simulink model "GuytonModel1986All_R2015a"  (R2015a)
settings: Solver=ode15s  StartTime=0  StopTime=383040  FixedStep=0.03  MaxStep=360  RelTol=1e-3
libraries: simulink x3
(part 3 of 5)

== system GuytonModel1986All_R2015a/Macula densa ==
  note: MACULA DENSA
  note: FNA
  note: NAPT1
  note: DAMPING
  CNA : Inport
  GFN : Inport  Port=2
  Constant1 : Constant
  Constant2 : Constant
  Constant3 : Constant
  Constant7 : Constant  Value=0.057
  GF2 : Constant  Value=0.1
  Integrator1 : Integrator  InitialConditionSource=external
  Product{2..3,7,15} (4 alike) : Product  SaturateOnIntegerOverflow=on  RndMeth=Zero  InputSameDT=on  OutDataTypeStr=Inherit: Same as first input
  RNAUGN : Constant  Value=5
  Sum3 : Sum  SaturateOnIntegerOverflow=on  InputSameDT=on  OutDataTypeStr=Inherit: Same as first input
  Sum30 : Sum  Inputs=+-  SaturateOnIntegerOverflow=on  InputSameDT=on  OutDataTypeStr=Inherit: Same as first input
  Sum9 : Sum  Inputs=-+  SaturateOnIntegerOverflow=on  InputSameDT=on  OutDataTypeStr=Inherit: Same as first input
  "upper limit 10 lower limit 0.3 " : Saturate  UpperLimit=10  LowerLimit=0.3  LinearizeAsGain=off
  upper limit 3.0 lower limit 0.1 : Saturate  UpperLimit=3  LowerLimit=0.1  LinearizeAsGain=off
  NAPT1 : Outport
  RNAUG1 : Outport  Port=2
  wires:
  Product15/1 -> Product3/1
  GFN/1 -> Product15/2
  CNA/1 -> Product15/1  "CNA"
  Constant7/1 -> Product3/2
  Product3/1 -> upper limit 3.0 lower limit 0.1/1  "NAPT"
  Constant1/1 -> Integrator1/2
  upper limit 3.0 lower limit 0.1/1 -> Sum9/2  "NAPT"
  GF2/1 -> Product7/2
  Sum9/1 -> Product7/1
  Product7/1 -> Integrator1/1
  Integrator1/1 -> Sum30/1, NAPT1/1, Sum9/1  "NAPT1"
  Constant2/1 -> Sum30/2
  Sum30/1 -> Product2/2
  RNAUGN/1 -> Product2/1
  Product2/1 -> Sum3/1
  Constant3/1 -> Sum3/2
  Sum3/1 -> "upper limit 10 lower limit 0.3 "/1
  "upper limit 10 lower limit 0.3 "/1 -> RNAUG1/1

== system GuytonModel1986All_R2015a/Muscle Local Blood Flow Control  ==
  note: Long term autoregulation
  note: Short term autoregulation
  note: AMM1
  note: if (POE<0.05) {POE=0.05}
  note: ARM
  note: Muscle Local Blood Flow Contro
  PMO : Inport
  A4K : Constant  Value=10
  A4K2 : Constant  Value=10000
  POK{1,4..5,10} (4 alike) : Constant
  POK15 : Constant  Value=0.3
  POK3 : Constant  Value=0.05
  POM : Constant  Value=0.2
  POM2 : Constant  Value=16
  PORM : Constant  Value=8
  Product : Product  SaturateOnIntegerOverflow=on  RndMeth=Zero  InputSameDT=on  OutDataTypeStr=Inherit: Same as first input
  Product1 : Product  Inputs=*/  SaturateOnIntegerOverflow=on  RndMeth=Zero  InputSameDT=on  OutDataTypeStr=Inherit: Same as first input
  Product5 : Product  SaturateOnIntegerOverflow=on  RndMeth=Zero  InputSameDT=on  OutDataTypeStr=Inherit: Same as first input
  Product7 : Product  Inputs=*/  SaturateOnIntegerOverflow=on  RndMeth=Zero  InputSameDT=on  OutDataTypeStr=Inherit: Same as first input
  Product8 : Product  SaturateOnIntegerOverflow=on  RndMeth=Zero  InputSameDT=on  OutDataTypeStr=Inherit: Same as first input
  Sum1 : Sum  Inputs=++|  SaturateOnIntegerOverflow=on  InputSameDT=on  OutDataTypeStr=Inherit: Same as first input
  Sum3 : Sum  Inputs=-+|  SaturateOnIntegerOverflow=on  InputSameDT=on  OutDataTypeStr=Inherit: Same as first input
  Sum7 : Sum  Inputs=+-  SaturateOnIntegerOverflow=on  InputSameDT=on  OutDataTypeStr=Inherit: Same as first input
  Sum8 : Sum  Inputs=++|  SaturateOnIntegerOverflow=on  InputSameDT=on  OutDataTypeStr=Inherit: Same as first input
  Sum9 : Sum  Inputs=-+|  SaturateOnIntegerOverflow=on  InputSameDT=on  OutDataTypeStr=Inherit: Same as first input
  Switch3 : Switch  Threshold=0.3  SaturateOnIntegerOverflow=on  InputSameDT=on
  Switch5 : Switch  Threshold=0.05  SaturateOnIntegerOverflow=on  InputSameDT=on
  integrator POB1 : Integrator  InitialConditionSource=external  InitialCondition=0.6577
  integrator POB4 : Integrator  InitialConditionSource=external  InitialCondition=0.6577
  " AMM" : Outport
  wires:
  Sum7/1 -> Product5/1, Product/1  "PDO"
  Sum8/1 -> Switch3/1, Switch3/2  "POF"
  Switch3/1 -> Sum9/2
  POK15/1 -> Switch3/3
  A4K2/1 -> Product7/2
  Sum9/1 -> Product7/1
  Product7/1 -> integrator POB4/1  "(POF-AMM2)/A4K2"
  POK10/1 -> integrator POB4/2
  integrator POB4/1 -> Sum9/1, Product8/1  "AMM2"
  POK5/1 -> Sum8/1
  Product5/1 -> Sum8/2
  POM2/1 -> Product5/2
  Product8/1 -> " AMM"/1
  Product1/1 -> integrator POB1/1  "(POE-AMM1)/A4K"
  A4K/1 -> Product1/2
  Sum3/1 -> Product1/1
  integrator POB1/1 -> Product8/2, Sum3/1  "AMM1"
  Switch5/1 -> Sum3/2  "POE"
  POK4/1 -> integrator POB1/2
  POK3/1 -> Switch5/3
  Sum1/1 -> Switch5/1, Switch5/2  "POE"
  POK1/1 -> Sum1/1
  Product/1 -> Sum1/2
  POM/1 -> Product/2
  PORM/1 -> Sum7/2
  PMO/1 -> Sum7/1

== system GuytonModel1986All_R2015a/Myogenic Autoregulation ==
  note: PA+PC
  note: PDIFF
  note: PADAPT
  note: PDIFF
  note: PADAPT
  note: Myogenic Autoregulation
  PA : Inport
  PC : Inport  Port=2
  MYOGTAU : Inport  Port=3
  TENSGN : Inport  Port=4
  Add25 : Sum
  Constant1 : Constant  Value=117
  Derivative : Derivative
  Integrator1 : Integrator  InitialConditionSource=external
  RAPDel=RAP-RAPAdp : Sum  Inputs=+-  SaturateOnIntegerOverflow=on  InputSameDT=on  OutDataTypeStr=Inherit: Same as first input
  RAPdot=RAPdel/AffTau : Product  Inputs=*/  SaturateOnIntegerOverflow=on  InputSameDT=on  OutDataTypeStr=Inherit: Same as first input
  RAPdot=RAPdel/AffTau1 : Product  Inputs=*/  SaturateOnIntegerOverflow=on  InputSameDT=on  OutDataTypeStr=Inherit: Same as first input
  RAPdot=RAPdel/AffTau2 : Product  Inputs=**  SaturateOnIntegerOverflow=on  InputSameDT=on  OutDataTypeStr=Inherit: Same as first input
  "[X,Y,Slope...]  - data from Coleman (1992)" : Constant  Value=[-30.0,1.5,0.0,0.0,1.0,-0.02,80.0,0.5,0.0]
  function MyogenResp(PDIFF) - spline interpolation : Subsystem  TreatAsAtomicUnit=on
      mask help: CURVILINEAR
      mask Help: Interpolates function value using  linear (if x<=0 or x>=x2) or cubic spline (if x0>x<x2) interpolation
      mask Display:
      | disp('C U R V I L I N E A R\n\nInterpolates function value \nusing  linear (if x<=0 or x>=x2)
      | \nor cubic spline (if x0>x<x2) interpolation\n\nINPUTS :\nx  -  value of independent variable\n xySlope - vector of coordinates and slope of 3 knots:\n[x0, y0, slope0,\n n1, y1, slope1,\n x2, y2, slope2]\n\nOUTPUTS :\ny - interpolated function value')
  MYOGRS : Outport
  wires:
  Constant1/1 -> Integrator1/2
  RAPdot=RAPdel/AffTau2/1 -> function MyogenResp(PDIFF) - spline interpolation/1(x)
  Derivative/1 -> RAPdot=RAPdel/AffTau2/1
  RAPdot=RAPdel/AffTau1/1 -> MYOGRS/1
  MYOGTAU/1 -> RAPdot=RAPdel/AffTau2/2, RAPdot=RAPdel/AffTau/2  "MYOGTAU"
  Integrator1/1 -> Derivative/1, RAPDel=RAP-RAPAdp/2
  RAPDel=RAP-RAPAdp/1 -> RAPdot=RAPdel/AffTau/1  "RAPDel"
  "[X,Y,Slope...]  - data from Coleman (1992)"/1 -> function MyogenResp(PDIFF) - spline interpolation/2(xySlope)
  RAPdot=RAPdel/AffTau/1 -> Integrator1/1  "DPADAPT"
  PC/1 -> Add25/2
  PA/1 -> Add25/1
  Add25/1 -> RAPDel=RAP-RAPAdp/1
  TENSGN/1 -> RAPdot=RAPdel/AffTau1/1
  function MyogenResp(PDIFF) - spline interpolation/1(y) -> RAPdot=RAPdel/AffTau1/2

== system GuytonModel1986All_R2015a/Myogenic Autoregulation of Afferent Arteriole ==
  note: MYOGENIC AUTOREGULATION IN KIDNEY
  note: PAR
  note: PADAPT
  note: PDIFF
  note: PADAPT
  PAR : Inport
  MYOGTAU : Inport  Port=2
  TENSGN : Inport  Port=3
  Constant1 : Constant  Value=100
  Integrator1 : Integrator  InitialConditionSource=external
  RAPDel=RAP-RAPAdp : Sum  Inputs=+-  SaturateOnIntegerOverflow=on  InputSameDT=on  OutDataTypeStr=Inherit: Same as first input
  RAPdot=RAPdel/AffTau : Product  Inputs=*/  SaturateOnIntegerOverflow=on  InputSameDT=on  OutDataTypeStr=Inherit: Same as first input
  RAPdot=RAPdel/AffTau1 : Product  Inputs=*/  SaturateOnIntegerOverflow=on  InputSameDT=on  OutDataTypeStr=Inherit: Same as first input
  "[X,Y,Slope...]  - data from Coleman (1992)" : Constant  Value=[-30.0,1.5,0.0,0.0,1.0,-0.02,80.0,0.5,0.0]
  function MyogenResp(PDIFF) - spline interpolation : Subsystem  TreatAsAtomicUnit=on
      mask help: CURVILINEAR
      mask Help: Interpolates function value using  linear (if x<=0 or x>=x2) or cubic spline (if x0>x<x2) interpolation
      mask Display:
      | disp('C U R V I L I N E A R\n\nInterpolates function value \nusing  linear (if x<=0 or x>=x2)
      | \nor cubic spline (if x0>x<x2) interpolation\n\nINPUTS :\nx  -  value of independent variable\n xySlope - vector of coordinates and slope of 3 knots:\n[x0, y0, slope0,\n n1, y1, slope1,\n x2, y2, slope2]\n\nOUTPUTS :\ny - interpolated function value')
  MYOGRSAA : Outport
  wires:
  Constant1/1 -> Integrator1/2
  RAPdot=RAPdel/AffTau1/1 -> MYOGRSAA/1
  MYOGTAU/1 -> RAPdot=RAPdel/AffTau/2  "MYOGTAU"
  Integrator1/1 -> RAPDel=RAP-RAPAdp/2
  RAPDel=RAP-RAPAdp/1 -> RAPdot=RAPdel/AffTau/1, function MyogenResp(PDIFF) - spline interpolation/1(x)  "RAPDel"
  "[X,Y,Slope...]  - data from Coleman (1992)"/1 -> function MyogenResp(PDIFF) - spline interpolation/2(xySlope)
  RAPdot=RAPdel/AffTau/1 -> Integrator1/1  "DPADAPT"
  PAR/1 -> RAPDel=RAP-RAPAdp/1
  TENSGN/1 -> RAPdot=RAPdel/AffTau1/1
  function MyogenResp(PDIFF) - spline interpolation/1(y) -> RAPdot=RAPdel/AffTau1/2

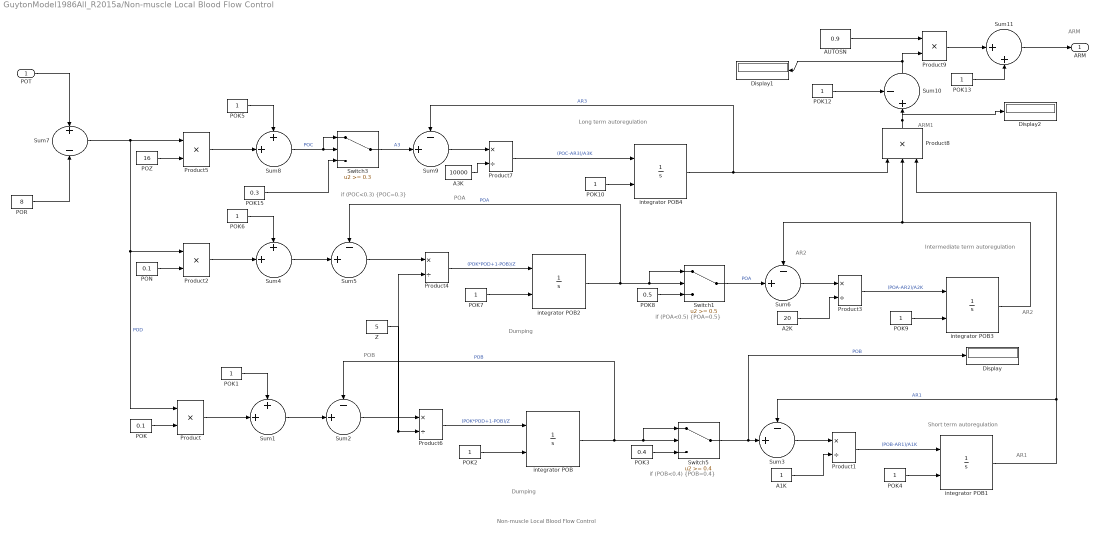
== system GuytonModel1986All_R2015a/Non-muscle Local Blood Flow Control  ==
  note: Long term autoregulation
  note: Intermediate term autoregulation
  note: Short term autoregulation
  note: Dumping
  note: Dumping
  note: ARM1
  note: if (POC<0.3) {POC=0.3}
  note: AR2
  note: AR2
  note: if (POA<0.5) {POA=0.5}
  note: POA
  note: AR1
  note: if (POB<0.4) {POB=0.4}
  note: POB
  note: ARM
  note: Non-muscle Local Blood Flow Control
  POT : Inport
  A1K : Constant
  A2K : Constant  Value=20
  A3K : Constant  Value=10000
  AUTOSN : Constant  Value=0.9
  Display : Display
  Display1 : Display
  Display2 : Display
  POK : Constant  Value=0.1
  POK{1..2,4..7,9..10,12..13} (10 alike) : Constant
  POK15 : Constant  Value=0.3
  POK3 : Constant  Value=0.4
  POK8 : Constant  Value=0.5
  PON : Constant  Value=0.1
  POR : Constant  Value=8
  POZ : Constant  Value=16
  Product{,2,5,9} (4 alike) : Product  SaturateOnIntegerOverflow=on  RndMeth=Zero  InputSameDT=on  OutDataTypeStr=Inherit: Same as first input
  Product{1,3..4,6..7} (5 alike) : Product  Inputs=*/  SaturateOnIntegerOverflow=on  RndMeth=Zero  InputSameDT=on  OutDataTypeStr=Inherit: Same as first input
  Product8 : Product  Inputs=3  SaturateOnIntegerOverflow=on  RndMeth=Zero  InputSameDT=on  OutDataTypeStr=Inherit: Same as first input
  Sum1 : Sum  Inputs=++|  SaturateOnIntegerOverflow=on  InputSameDT=on  OutDataTypeStr=Inherit: Same as first input
  Sum{2..3,5..6,9..10} (6 alike) : Sum  Inputs=-+|  SaturateOnIntegerOverflow=on  InputSameDT=on  OutDataTypeStr=Inherit: Same as first input
  Sum11 : Sum  Inputs=|++  SaturateOnIntegerOverflow=on  InputSameDT=on  OutDataTypeStr=Inherit: Same as first input
  Sum4 : Sum  Inputs=++|  SaturateOnIntegerOverflow=on  InputSameDT=on  OutDataTypeStr=Inherit: Same as first input
  Sum7 : Sum  Inputs=+-  SaturateOnIntegerOverflow=on  InputSameDT=on  OutDataTypeStr=Inherit: Same as first input
  Sum8 : Sum  Inputs=++|  SaturateOnIntegerOverflow=on  InputSameDT=on  OutDataTypeStr=Inherit: Same as first input
  Switch1 : Switch  Threshold=0.5  SaturateOnIntegerOverflow=on  InputSameDT=on
  Switch3 : Switch  Threshold=0.3  SaturateOnIntegerOverflow=on  InputSameDT=on
  Switch5 : Switch  Threshold=0.4  SaturateOnIntegerOverflow=on  InputSameDT=on
  Z : Constant  Value=5
  integrator POB{,1..4} (5 alike) : Integrator  InitialConditionSource=external  InitialCondition=0.6577
  " ARM" : Outport
  wires:
  Switch3/1 -> Sum9/2  "A3"
  POK15/1 -> Switch3/3
  Sum8/1 -> Switch3/1, Switch3/2  "POC"
  Sum11/1 -> " ARM"/1
  POK13/1 -> Sum11/2
  Product9/1 -> Sum11/1
  Sum10/1 -> Product9/2, Display1/1
  AUTOSN/1 -> Product9/1
  POK12/1 -> Sum10/1
  Product8/1 -> Sum10/2, Display2/1
  A3K/1 -> Product7/2
  Sum9/1 -> Product7/1
  Product7/1 -> integrator POB4/1  "(POC-AR3)/A3K"
  POK10/1 -> integrator POB4/2
  integrator POB4/1 -> Sum9/1, Product8/1  "AR3"
  POK5/1 -> Sum8/1
  Product5/1 -> Sum8/2
  POZ/1 -> Product5/2
  Product3/1 -> integrator POB3/1  "(POA-AR2)/A2K"
  A2K/1 -> Product3/2
  Sum6/1 -> Product3/1
  integrator POB3/1 -> Product8/2, Sum6/1
  Switch1/1 -> Sum6/2  "POA"
  POK9/1 -> integrator POB3/2
  POK8/1 -> Switch1/3
  Product4/1 -> integrator POB2/1  "(POK*POD+1-POB)/Z"
  Sum5/1 -> Product4/1
  integrator POB2/1 -> Sum5/1, Switch1/2, Switch1/1  "POA"
  Sum4/1 -> Sum5/2
  POK7/1 -> integrator POB2/2
  POK6/1 -> Sum4/1
  Product2/1 -> Sum4/2
  PON/1 -> Product2/2
  Product1/1 -> integrator POB1/1  "(POB-AR1)/A1K"
  A1K/1 -> Product1/2
  Sum3/1 -> Product1/1
  integrator POB1/1 -> Product8/3, Sum3/1  "AR1"
  Switch5/1 -> Sum3/2, Display/1  "POB"
  POK4/1 -> integrator POB1/2
  POK3/1 -> Switch5/3
  Product6/1 -> integrator POB/1  "(POK*POD+1-POB)/Z"
  Z/1 -> Product4/2, Product6/2
  Sum2/1 -> Product6/1
  integrator POB/1 -> Switch5/1, Switch5/2, Sum2/1  "POB"
  Sum1/1 -> Sum2/2
  POK2/1 -> integrator POB/2
  POK1/1 -> Sum1/1
  Product/1 -> Sum1/2
  POK/1 -> Product/2
  Sum7/1 -> Product5/1, Product2/1, Product/1  "POD"
  POR/1 -> Sum7/2
  POT/1 -> Sum7/1

== system GuytonModel1986All_R2015a/Peritubular Capillaries ==
  note: PERITUBULAR CAPILLARIES
  RFN : Inport
  GLPC : Inport  Port=2
  Constant1 : Constant  Value=1.0
  Constant13 : Constant  Value=1.2
  Constant2 : Constant  Value=1.0
  Constant3 : Constant  Value=1.0
  Integrator3 : Integrator  InitialConditionSource=external
  Product{1..3,5..6,14} (6 alike) : Product  SaturateOnIntegerOverflow=on  RndMeth=Zero  InputSameDT=on  OutDataTypeStr=Inherit: Same as first input
  Product4 : Product  Inputs=*/  SaturateOnIntegerOverflow=on  RndMeth=Zero  InputSameDT=on  OutDataTypeStr=Inherit: Same as first input
  RABSC : Constant  Value=0.5
  RFABD : Constant
  RFABM : Constant  Value=0.3
  RFABX : Constant  Value=0.8
  RFNM : Constant  Value=0.0
  RTPPR : Constant  Value=0.8999
  RTPPRS : Constant  Value=15.19999
  RTSPR : Constant  Value=6
  RVRS : Constant  Value=19.1669
  Sum1 : Sum  SaturateOnIntegerOverflow=on  InputSameDT=on  OutDataTypeStr=Inherit: Same as first input
  Sum12 : Sum  Inputs=-+  SaturateOnIntegerOverflow=on  InputSameDT=on  OutDataTypeStr=Inherit: Same as first input
  Sum2 : Sum  Inputs=+-  SaturateOnIntegerOverflow=on  InputSameDT=on  OutDataTypeStr=Inherit: Same as first input
  Sum3 : Sum  Inputs=--++  SaturateOnIntegerOverflow=on  InputSameDT=on  OutDataTypeStr=Inherit: Same as first input
  Sum4 : Sum  Inputs=+-  SaturateOnIntegerOverflow=on  InputSameDT=on  OutDataTypeStr=Inherit: Same as first input
  Sum5 : Sum  Inputs=-+  SaturateOnIntegerOverflow=on  InputSameDT=on  OutDataTypeStr=Inherit: Same as first input
  Sum6 : Sum  Inputs=+++  SaturateOnIntegerOverflow=on  InputSameDT=on  OutDataTypeStr=Inherit: Same as first input
  lower limit =0.0001 : Saturate  UpperLimit=inf  LowerLimit=0.0001  LinearizeAsGain=off
  lower limit =1.0 : Saturate  UpperLimit=inf  LowerLimit=1.0  LinearizeAsGain=off
  RFAB : Outport
  RCPRS : Outport  Port=2
  wires:
  RFN/1 -> Sum12/2
  Constant13/1 -> Sum12/1, Sum1/1
  Sum12/1 -> Product14/1, Product6/1
  RFABX/1 -> Product14/2
  Product14/1 -> Sum1/2
  RVRS/1 -> Product1/2
  Sum1/1 -> Product1/1
  Product1/1 -> Sum3/1, RCPRS/1  "RCPRS"
  RTPPRS/1 -> Sum2/2
  Product2/1 -> Sum2/1
  Sum2/1 -> lower limit =1.0/1
  lower limit =1.0/1 -> Sum3/2  "RTSPPC"
  RTPPR/1 -> Product2/1
  GLPC/1 -> Product2/2, Sum3/3
  RTSPR/1 -> Sum3/4
  RABSC/1 -> Product3/1
  Sum3/1 -> Product3/2  "RABSPR"
  Product3/1 -> Sum4/1  "RFAB1"
  Sum4/1 -> Product4/1
  RFABD/1 -> Product4/2
  Product4/1 -> Integrator3/1  "DRFAB2"
  Integrator3/1 -> Sum5/2, Sum4/2  "RFAB2"
  Constant1/1 -> Sum5/1
  RFABM/1 -> Product5/1
  Sum5/1 -> Product5/2
  RFNM/1 -> Product6/2
  Product5/1 -> Sum6/3
  Product6/1 -> Sum6/2
  Constant2/1 -> Sum6/1
  Sum6/1 -> lower limit =0.0001/1
  lower limit =0.0001/1 -> RFAB/1
  Constant3/1 -> Integrator3/2

== system GuytonModel1986All_R2015a/Plasma Protein Dynamics ==
  note: CPP
  note: 2
      | PPC=0.28*CPP+0.0019*CPP
  note: CPP
  note: DLP
  note: Plasma Protein Dynamics
  VP : Inport
  VTCLP : Inport  Port=2
  DPL : Inport  Port=3
  CPI : Inport  Port=4
  LPPR : Inport  Port=5
  PPD : Inport  Port=6
  DPR : Inport  Port=7
  Add1 : Sum  Inputs=+-
  Add2 : Sum
  Add3 : Sum  Inputs=+-
  Add4 : Sum
  Add5 : Sum  Inputs=+-
  CPR : Constant  Value=40
  Constant1 : Constant  Value=0.28
  Constant2 : Constant  Value=0.0019
  Constant3 : Constant  Value=0.00104
  Constant4 : Constant  Value=0
  Constant5 : Constant  Value=8
  Integrator : Integrator  InitialConditionSource=external
  LPK : Constant  Value=0.27285E-13
  Math Function : Math  Operator=pow  SaturateOnIntegerOverflow=on
  Math Function2 : Math  Operator=square  SaturateOnIntegerOverflow=on
  PRP0 : Constant  Value=216
  Product{1..2,4..6} (5 alike) : Product  Inputs=**  RndMeth=Zero
  Product3 : Product  Inputs=*/  RndMeth=Zero
  Sum1 : Sum  Inputs=---++  SaturateOnIntegerOverflow=on  InputSameDT=on  OutDataTypeStr=Inherit: Same as first input
  "if (CPPD1<0)  {CPPD=0} else {CPPD=CPPD1}" : Switch
  PPC : Outport
  DPC : Outport  Port=2
  CPP : Outport  Port=3
  DLP : Outport  Port=4
  wires:
  Integrator/1 -> Product3/1  "PRP"
  PRP0/1 -> Integrator/2
  VP/1 -> Product3/2  "VP"
  Product3/1 -> Math Function2/1, Product5/2, Product1/2, Add1/1, Add3/1, CPP/1
  Constant1/1 -> Product5/1
  Product5/1 -> Add4/1
  Math Function2/1 -> Product6/1
  Constant2/1 -> Product6/2
  Product6/1 -> Add4/2
  Add4/1 -> PPC/1  "PPC"
  VTCLP/1 -> Product1/1
  Product1/1 -> Add2/1  "PLPRL"
  CPI/1 -> Add1/2
  Add1/1 -> Product2/1
  Constant3/1 -> Product2/2
  Product2/1 -> Add2/2  "PLPRDF"
  Add2/1 -> DPC/1, Sum1/3  "DPC"
  CPR/1 -> Add3/2
  Add3/1 -> "if (CPPD1<0)  {CPPD=0} else {CPPD=CPPD1}"/1, "if (CPPD1<0)  {CPPD=0} else {CPPD=CPPD1}"/2  "CPPD1"
  Constant4/1 -> "if (CPPD1<0)  {CPPD=0} else {CPPD=CPPD1}"/3
  "if (CPPD1<0)  {CPPD=0} else {CPPD=CPPD1}"/1 -> Math Function/1  "CPPD"
  LPK/1 -> Product4/1
  Constant5/1 -> Math Function/2  "v"
  Math Function/1 -> Product4/2
  Product4/1 -> Add5/2  "LPPRDS"
  LPPR/1 -> Add5/1
  Add5/1 -> DLP/1, Sum1/5
  DPL/1 -> Sum1/4
  PPD/1 -> Sum1/2
  DPR/1 -> Sum1/1
  Sum1/1 -> Integrator/1  "DLP"

== system GuytonModel1986All_R2015a/Potassium Excretion ==
  note: POTASSIUM EXCRETION
  note: DAMPING
  CKE : Inport
  CNA : Inport  Port=2
  NADT : Inport  Port=3
  DTNAI : Inport  Port=4
  ANM : Inport  Port=5
  AMK : Inport  Port=6
  RFAB : Inport  Port=7
  REK : Inport  Port=8
  VUDN : Inport  Port=9
  ANMKEM : Constant  Value=2
  CKEEX1 : Constant  Value=4
  CKENORM1 : Constant  Value=5
  Constant{1..2,4,12..13} (5 alike) : Constant
  Constant11 : Constant  Value=0.00000001
  Constant3 : Constant  Value=0.0002275
  Display3 : Display
  Gain1 : Gain  Gain=0.000293  SaturateOnIntegerOverflow=on  OutDataTypeStr=Inherit: Same as input  ParamDataTypeStr=Inherit: Same as input
  Gain7 : Gain  Gain=0.06  SaturateOnIntegerOverflow=on  OutDataTypeStr=Inherit: Same as input  ParamDataTypeStr=Inherit: Same as input
  Integrator3 : Integrator  InitialConditionSource=external
  KDMP : Constant  Value=3
  Math Function2 : Math  Operator=pow  SaturateOnIntegerOverflow=on
  NADTKM : Constant  Value=0.5
  Product{1..2,5,14} (4 alike) : Product  SaturateOnIntegerOverflow=on  RndMeth=Zero  InputSameDT=on  OutDataTypeStr=Inherit: Same as first input
  Product11 : Product  Inputs=*/  SaturateOnIntegerOverflow=on  RndMeth=Zero  InputSameDT=on  OutDataTypeStr=Inherit: Same as first input
  Product13 : Product  Inputs=*/*  SaturateOnIntegerOverflow=on  RndMeth=Zero  InputSameDT=on  OutDataTypeStr=Inherit: Same as first input
  Product3 : Product  Inputs=***/  SaturateOnIntegerOverflow=on  RndMeth=Zero  InputSameDT=on  OutDataTypeStr=Inherit: Same as first input
  Product4 : Product  Inputs=*/  SaturateOnIntegerOverflow=on  RndMeth=Zero  InputSameDT=on  OutDataTypeStr=Inherit: Same as first input
  Product6 : Product  Inputs=*/  SaturateOnIntegerOverflow=on  RndMeth=Zero  InputSameDT=on  OutDataTypeStr=Inherit: Same as first input
  RFABKM : Constant  Value=0.03
  Sum1 : Sum  Inputs=-+  SaturateOnIntegerOverflow=on  InputSameDT=on  OutDataTypeStr=Inherit: Same as first input
  Sum11 : Sum  Inputs=+-  SaturateOnIntegerOverflow=on  InputSameDT=on  OutDataTypeStr=Inherit: Same as first input
  Sum12 : Sum  Inputs=-+  SaturateOnIntegerOverflow=on  InputSameDT=on  OutDataTypeStr=Inherit: Same as first input
  Sum13 : Sum  SaturateOnIntegerOverflow=on  InputSameDT=on  OutDataTypeStr=Inherit: Same as first input
  Sum2 : Sum  Inputs=-+  SaturateOnIntegerOverflow=on  InputSameDT=on  OutDataTypeStr=Inherit: Same as first input
  Sum3 : Sum  Inputs=++--  SaturateOnIntegerOverflow=on  InputSameDT=on  OutDataTypeStr=Inherit: Same as first input
  Sum4 : Sum  SaturateOnIntegerOverflow=on  InputSameDT=on  OutDataTypeStr=Inherit: Same as first input
  Sum5 : Sum  SaturateOnIntegerOverflow=on  InputSameDT=on  OutDataTypeStr=Inherit: Same as first input
  lower limit =0.1 : Saturate  UpperLimit=inf  LowerLimit=0.1  LinearizeAsGain=off
  lower limit =0.3 : Saturate  UpperLimit=inf  LowerLimit=0.3  LinearizeAsGain=off
  KODN : Outport
  KOD : Outport  Port=2
  CKU : Outport  Port=3
  wires:
  Sum5/1 -> lower limit =0.3/1
  Constant4/1 -> Sum5/1
  Product1/1 -> Sum5/2
  Integrator3/1 -> Sum11/2, Sum3/4  "DTKA"
  Constant3/1 -> Integrator3/2
  Sum4/1 -> Integrator3/1
  KDMP/1 -> Product11/2
  Product11/1 -> Sum4/1
  Constant11/1 -> Sum4/2
  Sum11/1 -> Product11/1
  Gain1/1 -> Sum11/1  "DTKA1"
  Product6/1 -> Gain1/1, CKU/1  "CKU"
  VUDN/1 -> Product6/2
  Product5/1 -> KOD/1
  REK/1 -> Product5/1
  Sum3/1 -> Product6/1, Product5/2, KODN/1  "KODN"
  Product13/1 -> Sum3/1  "DTKI"
  Product2/1 -> Sum3/3  "RFABK"
  RFABKM/1 -> Product2/1
  Sum2/1 -> Product2/2
  RFAB/1 -> Sum2/2
  Constant2/1 -> Sum2/1
  Gain7/1 -> Sum3/2  "DTKSC"
  Product3/1 -> Gain7/1
  Math Function2/1 -> Product3/2  "MCKE"
  lower limit =0.1/1 -> Product3/3  "NADTK"
  AMK/1 -> Product3/1
  DTNAI/1 -> Product13/1
  CKE/1 -> Product4/1, Product13/3  "CKE"
  CKEEX1/1 -> Math Function2/2  "v"
  Product4/1 -> Math Function2/1  "u"
  CKENORM1/1 -> Product4/2
  lower limit =0.3/1 -> Product3/4  "ANMKE"
  Sum1/1 -> Product1/2
  ANMKEM/1 -> Product1/1
  Constant1/1 -> Sum1/1
  ANM/1 -> Display3/1, Sum1/2
  NADT/1 -> Sum12/2
  CNA/1 -> Product13/2  "CNA"
  Sum12/1 -> Product14/2
  Constant12/1 -> Sum12/1
  NADTKM/1 -> Product14/1
  Product14/1 -> Sum13/2
  Constant13/1 -> Sum13/1
  Sum13/1 -> lower limit =0.1/1

== system GuytonModel1986All_R2015a/Pulmonary Fluid Dynamics ==
  note: PPN
  note: Pulmonary Fluid Dynamics
  PPA : Inport
  PLA : Inport  Port=2
  PPC : Inport  Port=3
  CPP : Inport  Port=4
  CPF : Inport  Port=5
  Con : Constant  Value=2
  Con1 : Constant  Value=11
  Constant9 : Constant  Value=0.150
  Gain1 : Gain  Gain=0.45  SaturateOnIntegerOverflow=on  OutDataTypeStr=Inherit: Same as input  ParamDataTypeStr=Inherit: Same as input
  Gain2 : Gain  Gain=0.55  SaturateOnIntegerOverflow=on  OutDataTypeStr=Inherit: Same as input  ParamDataTypeStr=Inherit: Same as input
  Gain3 : Gain  Gain=0.000225  SaturateOnIntegerOverflow=on  OutDataTypeStr=Inherit: Same as input  ParamDataTypeStr=Inherit: Same as input
  Gain4 : Gain  Gain=0.0003  SaturateOnIntegerOverflow=on  OutDataTypeStr=Inherit: Same as input  ParamDataTypeStr=Inherit: Same as input
  Gain5 : Gain  Gain=0.4  SaturateOnIntegerOverflow=on  OutDataTypeStr=Inherit: Same as input  ParamDataTypeStr=Inherit: Same as input
  Integrator1 : Integrator  InitialConditionSource=external  InitialCondition=0.0122822  LimitOutput=on  LowerSaturationLimit=0
  Integrator2 : Integrator  InitialConditionSource=external  InitialCondition=0.4296
  PPR0 : Constant  Value=0.4296
  Product : Product  Inputs=*/  SaturateOnIntegerOverflow=on  RndMeth=Zero  InputSameDT=on  OutDataTypeStr=Inherit: Same as first input
  Product1 : Product  SaturateOnIntegerOverflow=on  RndMeth=Zero  InputSameDT=on  OutDataTypeStr=Inherit: Same as first input
  Product2 : Product  SaturateOnIntegerOverflow=on  RndMeth=Zero  InputSameDT=on  OutDataTypeStr=Inherit: Same as first input
  Product5 : Product  Inputs=*/  SaturateOnIntegerOverflow=on  RndMeth=Zero  InputSameDT=on  OutDataTypeStr=Inherit: Same as first input
  Sum10 : Sum  SaturateOnIntegerOverflow=on  InputSameDT=on  OutDataTypeStr=Inherit: Same as first input
  Sum{4..5,9,11} (4 alike) : Sum  Inputs=+-  SaturateOnIntegerOverflow=on  InputSameDT=on  OutDataTypeStr=Inherit: Same as first input
  Sum2 : Sum  SaturateOnIntegerOverflow=on  InputSameDT=on  OutDataTypeStr=Inherit: Same as first input
  Sum3 : Sum  Inputs=-++-  SaturateOnIntegerOverflow=on  InputSameDT=on  OutDataTypeStr=Inherit: Same as first input
  VPF0 : Constant  Value=0.0122822
  DFP : Outport
  VPF : Outport  Port=2
  PCP : Outport  Port=3
  POS : Outport  Port=4
  PPI : Outport  Port=5
  PFI : Outport  Port=6
  PLF : Outport  Port=7
  CPN : Outport  Port=8
  PPN : Outport  Port=9
  PPR : Outport  Port=10
  PPD : Outport  Port=11
  wires:
  PPR0/1 -> Integrator2/2
  Sum11/1 -> Integrator2/1, PPD/1  "PPD"
  Integrator2/1 -> PPR/1, Product5/1  "PPR"
  Sum10/1 -> Gain4/1
  VPF0/1 -> Integrator1/2
  Sum5/1 -> Integrator1/1, DFP/1  "DFP"
  Integrator1/1 -> Product/2, Product5/2, VPF/1  "VPF"
  Gain4/1 -> PLF/1, Product2/2, Sum5/2  "PLF"
  PPA/1 -> Gain1/1
  PLA/1 -> Gain2/1
  Gain2/1 -> Sum2/2
  Gain1/1 -> Sum2/1
  PPC/1 -> Sum3/1
  CPF/1 -> Product1/1
  Product1/1 -> PFI/1, Sum5/1  "PFI"
  Constant9/1 -> Product/1
  Product/1 -> Sum9/2
  Con/1 -> Sum9/1
  Con1/1 -> Sum10/1
  CPP/1 -> Sum4/1
  Sum4/1 -> Gain3/1
  Gain5/1 -> POS/1, Sum3/3  "POS"
  Sum2/1 -> PCP/1, Sum3/2  "PCP"
  Sum9/1 -> PPI/1, Sum3/4, Sum10/2  "PPI"
  Sum3/1 -> Product1/2  "PGRPCM"
  Product5/1 -> CPN/1, Sum4/2, Gain5/1, Product2/1  "CPN"
  Product2/1 -> Sum11/2  "PPO"
  Gain3/1 -> PPN/1, Sum11/1

== system GuytonModel1986All_R2015a/Pulmonary O2 Delivery ==
  note: Pulmonary O2 Delivery
  VPF : Inport
  DOB : Inport  Port=2
  RMO : Inport  Port=3
  PO2DEF : Inport  Port=4
  PO2AMB : Inport  Port=5
  HM : Inport  Port=6
  Constant13 : Constant  Value=0.006
  Constant14 : Constant  Value=0.6
  Constant17 : Constant  Value=100
  Constant18 : Constant  Value=0.9775
  Gain6 : Gain  Gain=0.0266667  SaturateOnIntegerOverflow=on  OutDataTypeStr=Inherit: Same as input  ParamDataTypeStr=Inherit: Same as input
  Gain7 : Gain  Gain=5  SaturateOnIntegerOverflow=on  OutDataTypeStr=Inherit: Same as input  ParamDataTypeStr=Inherit: Same as input
  Product3 : Product  Inputs=3  SaturateOnIntegerOverflow=on  RndMeth=Zero  InputSameDT=on  OutDataTypeStr=Inherit: Same as first input
  Product4 : Product  SaturateOnIntegerOverflow=on  RndMeth=Zero  InputSameDT=on  OutDataTypeStr=Inherit: Same as first input
  Product6 : Product  Inputs=*/  SaturateOnIntegerOverflow=on  RndMeth=Zero  InputSameDT=on  OutDataTypeStr=Inherit: Same as first input
  Product7 : Product  Inputs=*/  SaturateOnIntegerOverflow=on  RndMeth=Zero  InputSameDT=on  OutDataTypeStr=Inherit: Same as first input
  Sum15 : Sum  SaturateOnIntegerOverflow=on  InputSameDT=on  OutDataTypeStr=Inherit: Same as first input
  Sum16 : Sum  SaturateOnIntegerOverflow=on  InputSameDT=on  OutDataTypeStr=Inherit: Same as first input
  Sum17 : Sum  Inputs=-+  SaturateOnIntegerOverflow=on  InputSameDT=on  OutDataTypeStr=Inherit: Same as first input
  Switch6 : Switch  Threshold=0.9775  SaturateOnIntegerOverflow=on  InputSameDT=on
  OSA : Outport
  OVA : Outport  Port=2
  wires:
  HM/1 -> Product4/2
  VPF/1 -> Sum16/1
  DOB/1 -> Sum15/1
  RMO/1 -> Sum15/2
  Constant13/1 -> Sum16/2
  Sum16/1 -> Product3/1
  Sum15/1 -> Product3/2
  Constant14/1 -> Product3/3
  Product3/1 -> Gain6/1
  Gain6/1 -> Product6/1
  PO2DEF/1 -> Product6/2
  Product6/1 -> Sum17/1
  PO2AMB/1 -> Sum17/2
  Sum17/1 -> Product7/1
  Constant17/1 -> Product7/2
  Product7/1 -> Switch6/3, Switch6/2
  Constant18/1 -> Switch6/1
  Gain7/1 -> Product4/1
  Switch6/1 -> OSA/1, Gain7/1
  Product4/1 -> OVA/1

== system GuytonModel1986All_R2015a/Red cells production and destruction ==
  note: VIM
  note: VB
  note: VRC
  note: RC2
  note: VP
  note: HM
  note: OSA
  note: REK
  note: RFN
  note: RC1
  note: RC2
  note: Red cells production and destruction
  OSA : Inport
  VP : Inport  Port=2
  VIM : Inport  Port=3
  RFN : Inport  Port=4
  REK : Inport  Port=5
  Constant1 : Constant  Value=0.97
  Constant2 : Constant  Value=0.9
  Constant3 : Constant  Value=1.0
  Constant4 : Constant  Value=0.0005568
  Constant5 : Constant  Value=0.00014
  Constant7 : Constant  Value=0.000004
  Gain2 : Gain  Gain=100  SaturateOnIntegerOverflow=on  OutDataTypeStr=Inherit: Same as input  ParamDataTypeStr=Inherit: Same as input
  Product : Product  Inputs=*/  SaturateOnIntegerOverflow=on  RndMeth=Zero  InputSameDT=on  OutDataTypeStr=Inherit: Same as first input
  Product1 : Product  SaturateOnIntegerOverflow=on  RndMeth=Zero  InputSameDT=on  OutDataTypeStr=Inherit: Same as first input
  Product2 : Product  Inputs=**/  SaturateOnIntegerOverflow=on  RndMeth=Zero  InputSameDT=on  OutDataTypeStr=Inherit: Same as first input
  Product3 : Product  Inputs=3  SaturateOnIntegerOverflow=on  RndMeth=Zero  InputSameDT=on  OutDataTypeStr=Inherit: Same as first input
  Product4 : Product  SaturateOnIntegerOverflow=on  RndMeth=Zero  InputSameDT=on  OutDataTypeStr=Inherit: Same as first input
  Product5 : Product  SaturateOnIntegerOverflow=on  RndMeth=Zero  InputSameDT=on  OutDataTypeStr=Inherit: Same as first input
  RKC : Constant  Value=0.0000058
  Sum1 : Sum  Inputs=+-  SaturateOnIntegerOverflow=on  InputSameDT=on  OutDataTypeStr=Inherit: Same as first input
  Sum2 : Sum  SaturateOnIntegerOverflow=on  InputSameDT=on  OutDataTypeStr=Inherit: Same as first input
  Sum6 : Sum  Inputs=-+  SaturateOnIntegerOverflow=on  InputSameDT=on  OutDataTypeStr=Inherit: Same as first input
  Sum7 : Sum  SaturateOnIntegerOverflow=on  InputSameDT=on  OutDataTypeStr=Inherit: Same as first input
  Switch1 : Switch  Threshold=0.00014  SaturateOnIntegerOverflow=on  InputSameDT=on
  Switch2 : Switch  Threshold=0.000004  SaturateOnIntegerOverflow=on  InputSameDT=on
  "VRC " : Integrator  InitialConditionSource=external  InitialCondition=2.00151
  VRCinit : Constant  Value=2
  VRC : Outport
  VB : Outport  Port=2
  HM : Outport  Port=3
  RC1 : Outport  Port=4
  RC2 : Outport  Port=5
  wires:
  "VRC "/1 -> Sum7/1, Product/1, Product3/3, VRC/1  "VRC"
  Sum6/1 -> "VRC "/1
  Product/1 -> Gain2/1  "HM1"
  Sum7/1 -> Product/2, VB/1  "VB"
  VRCinit/1 -> "VRC "/2
  RKC/1 -> Product3/2
  VIM/1 -> Product3/1
  Product3/1 -> Sum6/1, RC2/1  "RC2"
  VP/1 -> Sum7/2
  Gain2/1 -> HM/1, Product5/2  "HM"
  Constant1/1 -> Sum1/1
  OSA/1 -> Sum1/2
  Sum1/1 -> Product1/1
  Constant2/1 -> Product1/2
  Product1/1 -> Sum2/1
  Constant3/1 -> Sum2/2
  Sum2/1 -> Product4/1
  Constant4/1 -> Product4/2
  Constant5/1 -> Switch1/1
  Switch1/1 -> Switch2/1, Switch2/2
  Constant7/1 -> Switch2/3
  Switch2/1 -> Sum6/2, RC1/1  "RC1"
  Product4/1 -> Product2/2
  REK/1 -> Product2/1
  Product5/1 -> Product2/3
  RFN/1 -> Product5/1
  Product2/1 -> Switch1/2, Switch1/3

== system GuytonModel1986All_R2015a/Renal Perfusion ==
  note: RENAL PERFUSION
  note: RFN
  note: RBF
  PA : Inport
  GBL : Inport  Port=2
  PVS : Inport  Port=3
  AAR : Inport  Port=4
  EAR : Inport  Port=5
  REK : Inport  Port=6
  Product1 : Product  SaturateOnIntegerOverflow=on  RndMeth=Zero  InputSameDT=on  OutDataTypeStr=Inherit: Same as first input
  Product2 : Product  Inputs=*/  SaturateOnIntegerOverflow=on  RndMeth=Zero  InputSameDT=on  OutDataTypeStr=Inherit: Same as first input
  Product4 : Product  Inputs=/*  SaturateOnIntegerOverflow=on  RndMeth=Zero  InputSameDT=on  OutDataTypeStr=Inherit: Same as first input
  Sum1 : Sum  Inputs=2  SaturateOnIntegerOverflow=on  InputSameDT=on  OutDataTypeStr=Inherit: Same as first input
  Sum2 : Sum  Inputs=+-  SaturateOnIntegerOverflow=on  InputSameDT=on  OutDataTypeStr=Inherit: Same as first input
  Sum3 : Sum  Inputs=+-  SaturateOnIntegerOverflow=on  InputSameDT=on  OutDataTypeStr=Inherit: Same as first input
  Sum4 : Sum  Inputs=+-  SaturateOnIntegerOverflow=on  InputSameDT=on  OutDataTypeStr=Inherit: Same as first input
  PAR : Outport
  RFN : Outport  Port=2
  RR : Outport  Port=3
  RBF : Outport  Port=4
  wires:
  Sum3/1 -> Product4/2
  Sum1/1 -> Product2/2  "IRR"
  Sum2/1 -> Product2/1
  PVS/1 -> Sum3/2, Sum2/2  "PVS"
  PA/1 -> Sum3/1, Sum4/1  "PA"
  GBL/1 -> Sum4/2  "GBL"
  Sum4/1 -> Sum2/1, PAR/1  "PAR"
  Product2/1 -> Product1/1, RFN/1
  REK/1 -> Product1/2
  Product1/1 -> Product4/1, RBF/1
  AAR/1 -> Sum1/1
  EAR/1 -> Sum1/2
  Product4/1 -> RR/1

== system GuytonModel1986All_R2015a/Resistances in the Pulmonary Circulation and Pulmonary Venous Pressure ==
  note: CPA
  note: Resistances in the Pulmonary Circulation and Pulmonary Venous Pressure
  PPA : Inport
  PLA : Inport  Port=2
  QPO : Inport  Port=3
  Add1 : Sum  Inputs=-+
  Add5 : Sum  Inputs=2
  Add6 : Sum
  CN4 : Constant  Value=0.00001
  CN5 : Constant  Value=20
  CPA=PP1^0.5 : Math  Operator=sqrt  SaturateOnIntegerOverflow=on
  Divide : Product  Inputs=/*
  Gain2 : Gain  Gain=0.026
  Gain3 : Gain  Gain=0.0357
  RPA=1/CPA : Math  Operator=reciprocal  SaturateOnIntegerOverflow=on
  RPV=1/CPV : Math  Operator=reciprocal  SaturateOnIntegerOverflow=on
  if PP1 < 0.00001 PP1=0.00001 : Switch  Threshold=0.00001
  RPA : Outport
  RPV : Outport  Port=2
  RPT : Outport  Port=3
  PVP : Outport  Port=4
  wires:
  Add1/1 -> PVP/1
  Divide/1 -> Add1/1
  QPO/1 -> Divide/2
  Add6/1 -> RPT/1
  RPV=1/CPV/1 -> Divide/1, RPV/1, Add6/2  "RPV"
  Gain3/1 -> RPV=1/CPV/1  "CPV"
  Add5/1 -> Gain3/1  "PL1"
  PLA/1 -> Add5/1
  CN5/1 -> Add5/2
  RPA=1/CPA/1 -> Add6/1, RPA/1
  CPA=PP1^0.5/1 -> RPA=1/CPA/1
  if PP1 < 0.00001 PP1=0.00001/1 -> CPA=PP1^0.5/1  "PP1"
  CN4/1 -> if PP1 < 0.00001 PP1=0.00001/3
  Gain2/1 -> if PP1 < 0.00001 PP1=0.00001/1, if PP1 < 0.00001 PP1=0.00001/2  "PP1"
  PPA/1 -> Add1/2, Gain2/1

== system GuytonModel1986All_R2015a/Resistances in the Systemic Circulation  ==
  note: RESISTANCES IN
      | THE SYSTEMIC CIRCULATION
  note: RSNV
  note: PA/PAnorm
  note: RSNA
  PA : Inport
  RAM : Inport  Port=2
  RAR : Inport  Port=3
  MYOGRS : Inport  Port=4
  AUM : Inport  Port=5
  VIM : Inport  Port=6
  ANU : Inport  Port=7
  AHMR : Inport  Port=8
  ATRRFB : Inport  Port=9
  AMM : Inport  Port=10
  ARM : Inport  Port=11
  RVSM : Inport  Port=12
  AVE : Inport  Port=13
  ANUVN : Inport  Port=14
  PC : Inport  Port=15
  (0.01*PA)^1.41 : Math  Operator=pow  SaturateOnIntegerOverflow=on
  Add1 : Sum  Inputs=+-
  Add2 : Sum  Inputs=|++
  Add25 : Sum
  Add3 : Sum  Inputs=-+|
  CN2 : Constant  Value=0.0212
  CN3 : Integrator  InitialConditionSource=external
  CN7 : Constant  Value=0.2
  Divide2 : Product  Inputs=4
  Divide3 : Product  Inputs=****//
  Divide4 : Product  Inputs=3
  Divide5 : Product
  Divide6 : Product
  Divide7 : Product  Inputs=*/
  Divide8 : Product  Inputs=4
  Divide9 : Product  Inputs=3
  Gain1 : Gain  Gain=0.1
  Gain5 : Gain  Gain=0.01
  PAEX : Constant  Value=1.41
  PAEX1 : Constant  Value=17
  PAEX2 : Constant  Value=0.3594
  PAEX5 : Constant  Value=1.79
  RSN : Outport
  RSM : Outport  Port=2
  RVS : Outport  Port=3
  wires:
  PC/1 -> Add1/1
  Add3/1 -> Gain1/1
  Gain1/1 -> CN3/1
  Add25/1 -> RSN/1
  Divide9/1 -> Add25/2
  MYOGRS/1 -> Divide9/2, Divide2/4  "MYOGRS"
  Divide8/1 -> Divide9/3, RVS/1  "RVS"
  RAM/1 -> Divide2/3
  AHMR/1 -> Divide3/3
  ANU/1 -> Divide3/2
  VIM/1 -> Divide3/4, Divide8/1  "VIM"
  Divide7/1 -> Divide8/2  "RV1"
  AVE/1 -> Divide8/3
  ANUVN/1 -> Divide8/4
  RVSM/1 -> Divide7/1
  CN3/1 -> Divide7/2, Add3/1  "CN3"
  Divide6/1 -> Add3/2
  CN2/1 -> Divide6/1
  Add2/1 -> Divide6/2
  Divide5/1 -> Add2/1
  CN7/1 -> Divide5/1
  Add1/1 -> Divide5/2
  PAEX1/1 -> Add2/2, Add1/2
  PAEX2/1 -> CN3/2
  ARM/1 -> Divide4/3
  Divide4/1 -> Add25/1
  RAR/1 -> Divide4/2
  Divide2/1 -> RSM/1  "RSM"
  AMM/1 -> Divide2/2
  Divide3/1 -> Divide4/1, Divide2/1  "R1"
  ATRRFB/1 -> Divide3/5
  AUM/1 -> Divide3/1
  (0.01*PA)^1.41/1 -> Divide3/6  "PAM"
  PAEX/1 -> (0.01*PA)^1.41/2  "PAEX"
  Gain5/1 -> (0.01*PA)^1.41/1
  PA/1 -> Gain5/1
  PAEX5/1 -> Divide9/1

== system GuytonModel1986All_R2015a/Right Heart Pumping ==
  note: Right Heart Pumping
  PRA : Inport
  PPA : Inport  Port=2
  AUH : Inport  Port=3
  OSA : Inport  Port=4
  HSR : Inport  Port=5
  HPR : Inport  Port=6
  HMD : Inport  Port=7
  QLO : Inport  Port=8
  QLN : Inport  Port=9
  Add1 : Sum  Inputs=2
  Add17 : Sum  Inputs=+-|
  Display1 : Display
  Display12 : Display
  Display4 : Display
  Divide1 : Product  Inputs=**
  Divide2 : Product  Inputs=*/
  Divide3 : Product  Inputs=6
  Divide4 : Product  Inputs=*/
  Divide5 : Product
  Divide7 : Product  Inputs=**
  QRF : Constant  Value=0.6
  VLAinit : Constant
  function StarlingRNorm(PLA) cubic spline interpolation x=[-6,-3,-1,0,2,4,8] y=[0,0.75,2.6,5.0,9.8,12.1,13.5] : Lookup_n-D  NumberOfTableDimensions=1  BreakpointsForDimension1=[-10,-9, -8,-7,-6, -3, -1, 2, 4, 8,8.5, 9,10,11,12,13]  Table=[0,0, 0,0,0,0.75,2.6,9.8,12.1,13.5,13.5,13.5,13.5,13.5,13.5,13.5]  InterpMethod=Cubic spline  ExtrapMethod=Clip  InputSameDT=on
  function rightHeartLoading(PP2) cubic spline interpolation x=[-0,-20,24,30,38,45] y=[1.06,0.97,0.93,0.8,0.46,0] : Lookup_n-D  NumberOfTableDimensions=1  BreakpointsForDimension1=[0,10,20, 24, 30, 38, 45]  Table=[1.06,1.03, 0.97,0.93,0.8,0.46,0]  InterpMethod=Cubic spline  ExtrapMethod=Clip  InputSameDT=on
  QRO : Outport
  QRN : Outport  Port=2
  RVM : Outport  Port=3
  wires:
  Divide7/1 -> QRO/1
  Add1/1 -> Divide7/2  "HPEF"
  Divide5/1 -> Display4/1, Add1/2
  Divide3/1 -> Display12/1, Add1/1
  Divide4/1 -> Divide5/2
  AUH/1 -> Divide3/3, Divide1/2
  OSA/1 -> Divide1/1
  QLO/1 -> Divide4/1
  QLN/1 -> Divide4/2
  HMD/1 -> Divide3/6
  HPR/1 -> Divide3/5
  HSR/1 -> Divide3/4
  Add17/1 -> Display1/1, Divide3/2
  function rightHeartLoading(PP2) cubic spline interpolation x=[-0,-20,24,30,38,45] y=[1.06,0.97,0.93,0.8,0.46,0]/1 -> RVM/1, Divide3/1  "RVM"
  Divide2/1 -> function rightHeartLoading(PP2) cubic spline interpolation x=[-0,-20,24,30,38,45] y=[1.06,0.97,0.93,0.8,0.46,0]/1  "PP2"
  PPA/1 -> Divide2/1
  Divide1/1 -> Divide2/2
  QRF/1 -> Divide5/1, Add17/2
  VLAinit/1 -> Add17/1
  function StarlingRNorm(PLA) cubic spline interpolation x=[-6,-3,-1,0,2,4,8] y=[0,0.75,2.6,5.0,9.8,12.1,13.5]/1 -> QRN/1, Divide7/1  "QRN"
  PRA/1 -> function StarlingRNorm(PLA) cubic spline interpolation x=[-6,-3,-1,0,2,4,8] y=[0,0.75,2.6,5.0,9.8,12.1,13.5]/1

== system GuytonModel1986All_R2015a/Sodium Excretion ==
  note: DAMPING
  note: DAMPING
  note: SODIUM EXCRETION
  note: lower limit
      | DTNARA=0.9999e-6
  note: Treshold=1
      | if (NADT1>Treshold) {NADT=NADT1}
      | else {NADT=NADT2}
  NAPT1 : Inport
  RFAB : Inport  Port=2
  VUDN : Inport  Port=3
  AMNA : Inport  Port=4
  AHM : Inport  Port=5
  REK : Inport  Port=6
  DIURET : Inport  Port=7
  AHMNAR : Constant  Value=0.3
  Constant10 : Constant  Value=0.4
  Constant11 : Constant  Value=100
  Constant{4..5,8..9} (4 alike) : Constant
  Constant6 : Constant  Value=2
  DTACN : Constant  Value=100
  DTNARN : Constant  Value=0.4
  GFR3 : Constant  Value=0.1
  Integrator2 : Integrator  InitialConditionSource=external  LimitOutput=on  LowerSaturationLimit=0.9999e-6
  Integrator3 : Integrator  InitialConditionSource=external
  Math Function : Math  Operator=pow  SaturateOnIntegerOverflow=on
  NADMP : Constant  Value=40
  NARSB1 : Constant  Value=16
  Product{2,5,10..11} (4 alike) : Product  Inputs=*/  SaturateOnIntegerOverflow=on  RndMeth=Zero  InputSameDT=on  OutDataTypeStr=Inherit: Same as first input
  Product{3..4,8..9,12} (5 alike) : Product  SaturateOnIntegerOverflow=on  RndMeth=Zero  InputSameDT=on  OutDataTypeStr=Inherit: Same as first input
  Product27 : Product  Inputs=****/  SaturateOnIntegerOverflow=on  RndMeth=Zero  InputSameDT=on  OutDataTypeStr=Inherit: Same as first input
  Sum10 : Sum  Inputs=+-  SaturateOnIntegerOverflow=on  InputSameDT=on  OutDataTypeStr=Inherit: Same as first input
  Sum11 : Sum  Inputs=-+  SaturateOnIntegerOverflow=on  InputSameDT=on  OutDataTypeStr=Inherit: Same as first input
  Sum4 : Sum  Inputs=+-  SaturateOnIntegerOverflow=on  InputSameDT=on  OutDataTypeStr=Inherit: Same as first input
  Sum5 : Sum  SaturateOnIntegerOverflow=on  InputSameDT=on  OutDataTypeStr=Inherit: Same as first input
  Sum6 : Sum  Inputs=+-  SaturateOnIntegerOverflow=on  InputSameDT=on  OutDataTypeStr=Inherit: Same as first input
  Sum7 : Sum  SaturateOnIntegerOverflow=on  InputSameDT=on  OutDataTypeStr=Inherit: Same as first input
  Sum8 : Sum  Inputs=-+  SaturateOnIntegerOverflow=on  InputSameDT=on  OutDataTypeStr=Inherit: Same as first input
  Switch16 : Switch  Threshold=1  SaturateOnIntegerOverflow=on  InputSameDT=on
  lower limit 0.00000001 : Saturate  UpperLimit=inf  LowerLimit=0.00000001  LinearizeAsGain=off
  NADT : Outport
  DTNAI : Outport  Port=2
  NODN : Outport  Port=3
  NOD : Outport  Port=4
  CNU : Outport  Port=5
  wires:
  VUDN/1 -> Product10/2
  Product12/1 -> NOD/1
  REK/1 -> Product12/2
  Product11/1 -> Integrator3/1
  NADMP/1 -> Product11/2
  Sum11/1 -> Product11/1
  Integrator3/1 -> Sum11/1, Product2/1  "DTNAC"
  Product10/1 -> CNU/1, Sum11/2  "CNU"
  lower limit 0.00000001/1 -> Product10/1, Product12/1, NODN/1  "NODN"
  Constant11/1 -> Integrator3/2
  Sum10/1 -> lower limit 0.00000001/1  "NODN"
  Product9/1 -> Integrator2/1
  Constant10/1 -> Integrator2/2
  GFR3/1 -> Product9/1
  Sum8/1 -> Product9/2
  Integrator2/1 -> Sum8/1, Sum10/2  "DTNARA"
  Product3/1 -> Sum8/2  "DTNAR1"
  Sum7/1 -> Product27/2
  Constant9/1 -> Sum7/1
  Product8/1 -> Sum7/2
  AHMNAR/1 -> Product8/1
  Sum6/1 -> Product8/2
  RFAB/1 -> Product27/1
  AMNA/1 -> Product27/3
  Product5/1 -> DTNAI/1, Sum10/1  "DTNAI"
  Constant6/1 -> Product5/2
  Switch16/1 -> NADT/1, Product5/1  "NADT"
  Math Function/1 -> Switch16/3  "NADT2"
  Sum5/1 -> Switch16/1, Switch16/2  "NADT1"
  Constant5/1 -> Sum5/2
  Product4/1 -> Sum5/1
  NARSB1/1 -> Math Function/2, Product4/2
  Sum4/1 -> Product4/1
  Constant4/1 -> Sum4/2
  NAPT1/1 -> Math Function/1, Sum4/1  "NAPT1"
  DTACN/1 -> Product2/2
  DIURET/1 -> Product27/5
  Product2/1 -> Product27/4  "DTNAC/NDTAC"
  AHM/1 -> Sum6/1
  Constant8/1 -> Sum6/2
  Product27/1 -> Product3/2  "MDTNAR"
  DTNARN/1 -> Product3/1

== system GuytonModel1986All_R2015a/Systemic Capillary Pressure ==
  note: Systemic Capillary Pressure
  PVS : Inport
  BFN : Inport  Port=2
  RVS : Inport  Port=3
  Add4 : Sum
  Divide1 : Product  Inputs=3
  PAEX4 : Constant  Value=1.79
  PC : Outport
  wires:
  RVS/1 -> Divide1/3
  PAEX4/1 -> Divide1/1
  BFN/1 -> Divide1/2
  Divide1/1 -> Add4/1
  Add4/1 -> PC/1
  PVS/1 -> Add4/2

== system GuytonModel1986All_R2015a/The control Functions of Aldosterone ==
  note: THE CONTROL FUNCTIONS OF ALDOSTERONE
  note: AMR
  note: AMC
  note: AM1
  ANM : Inport
  CKE : Inport  Port=2
  ALD : Inport  Port=3
  ALDMM : Constant  Value=6.0
  AMKM : Constant  Value=0.5
  AMKMUL : Constant  Value=12
  AMNAM : Constant  Value=1.2
  AMREX : Constant  Value=0.3
  AMT : Constant  Value=60
  ANMALM : Constant  Value=3
  Constant1 : Constant  Value=5
  Constant{2..11} (10 alike) : Constant
  Integrator3 : Integrator  InitialConditionSource=external
  Math Function2 : Math  Operator=pow  SaturateOnIntegerOverflow=on
  Product{1,3,5..7} (5 alike) : Product  SaturateOnIntegerOverflow=on  RndMeth=Zero  InputSameDT=on  OutDataTypeStr=Inherit: Same as first input
  Product2 : Product  Inputs=*/  SaturateOnIntegerOverflow=on  RndMeth=Zero  InputSameDT=on  OutDataTypeStr=Inherit: Same as first input
  Product4 : Product  Inputs=*/  SaturateOnIntegerOverflow=on  RndMeth=Zero  InputSameDT=on  OutDataTypeStr=Inherit: Same as first input
  Sum1 : Sum  SaturateOnIntegerOverflow=on  InputSameDT=on  OutDataTypeStr=Inherit: Same as first input
  Sum10 : Sum  Inputs=2  SaturateOnIntegerOverflow=on  InputSameDT=on  OutDataTypeStr=Inherit: Same as first input
  Sum18 : Sum  Inputs=+-  SaturateOnIntegerOverflow=on  InputSameDT=on  OutDataTypeStr=Inherit: Same as first input
  Sum2 : Sum  Inputs=-+  SaturateOnIntegerOverflow=on  InputSameDT=on  OutDataTypeStr=Inherit: Same as first input
  Sum3 : Sum  SaturateOnIntegerOverflow=on  InputSameDT=on  OutDataTypeStr=Inherit: Same as first input
  Sum4 : Sum  Inputs=-++  SaturateOnIntegerOverflow=on  InputSameDT=on  OutDataTypeStr=Inherit: Same as first input
  Sum5 : Sum  Inputs=-+  SaturateOnIntegerOverflow=on  InputSameDT=on  OutDataTypeStr=Inherit: Same as first input
  Sum6 : Sum  Inputs=2  SaturateOnIntegerOverflow=on  InputSameDT=on  OutDataTypeStr=Inherit: Same as first input
  Sum7 : Sum  Inputs=-+  SaturateOnIntegerOverflow=on  InputSameDT=on  OutDataTypeStr=Inherit: Same as first input
  Sum8 : Sum  Inputs=2  SaturateOnIntegerOverflow=on  InputSameDT=on  OutDataTypeStr=Inherit: Same as first input
  Sum9 : Sum  Inputs=+-  SaturateOnIntegerOverflow=on  InputSameDT=on  OutDataTypeStr=Inherit: Same as first input
  lower limit -0.2 : Saturate  UpperLimit=inf  LowerLimit=-0.2
  "lower limit 0 " : Saturate  UpperLimit=inf  LowerLimit=0
  "lower limit 0.2 " : Saturate  UpperLimit=inf  LowerLimit=0.2
  upper limit 15.0 lower limit 0.4 : Saturate  UpperLimit=15  LowerLimit=0.4
  AMK : Outport
  AMNA : Outport  Port=2
  AMC : Outport  Port=3
  wires:
  ANM/1 -> Sum18/1
  Constant8/1 -> Sum18/2
  Sum18/1 -> Product1/2
  ANMALM/1 -> Product1/1
  Product1/1 -> lower limit -0.2/1
  CKE/1 -> Sum1/2
  lower limit -0.2/1 -> Sum1/1
  Constant1/1 -> Product2/2
  Sum1/1 -> Product2/1
  Product2/1 -> Sum2/2
  Constant2/1 -> Sum2/1
  Sum2/1 -> Product3/2
  AMKMUL/1 -> Product3/1
  Constant3/1 -> Sum3/2
  Product3/1 -> Sum3/1
  Sum3/1 -> "lower limit 0 "/1
  "lower limit 0 "/1 -> Sum4/2  "AMR"
  Constant4/1 -> Integrator3/2
  ALD/1 -> Sum4/3
  AMT/1 -> Product4/2
  Sum4/1 -> Product4/1
  Product4/1 -> Integrator3/1
  Integrator3/1 -> Sum4/1, Math Function2/1, AMC/1  "u"
  AMREX/1 -> Math Function2/2  "v"
  Math Function2/1 -> Sum5/2
  Constant5/1 -> Sum5/1
  Sum5/1 -> Product5/2
  ALDMM/1 -> Product5/1
  Product5/1 -> Sum6/2
  Constant6/1 -> Sum6/1
  Sum6/1 -> Sum7/2, Sum9/1  "AM"
  Constant7/1 -> Sum7/1
  Sum7/1 -> Product6/2
  AMKM/1 -> Product6/1
  Product6/1 -> Sum8/2
  Constant9/1 -> Sum8/1
  Sum8/1 -> "lower limit 0.2 "/1
  "lower limit 0.2 "/1 -> AMK/1
  Constant10/1 -> Sum9/2
  Sum9/1 -> Product7/1
  AMNAM/1 -> Product7/2
  Product7/1 -> Sum10/1
  Constant11/1 -> Sum10/2
  Sum10/1 -> upper limit 15.0 lower limit 0.4/1
  upper limit 15.0 lower limit 0.4/1 -> AMNA/1
